simulink model "slo_flathier"  (R2015b)
settings: Solver=FixedStepDiscrete  SolverMode=SingleTasking  StartTime=0.0  StopTime=10  RelTol=1e-3
libraries: hdlsllib x1
CloseFcn:
  | rtwprivate ssgencode ModelCloseRequest Hysteresis_test1
settings Model: Creator=at-mt  LastModifiedBy=amatsumo
settings DataIOCC: SaveFormat=Array  SignalLoggingSaveFormat=ModelDataLogs  SaveOutput=off  SignalLogging=off  SaveTime=off
settings OptimizationCC: BlockReduction=off  ConditionallyExecuteInputs=off  DefaultParameterBehavior=Inlined  ExpressionDepthLimit=2147483647
settings DebuggingCC: AlgebraicLoopMsg=error  UnderspecifiedInitializationDetection=Classic  MergeDetectMultiDrivingBlocksExec=none  SolverPrmCheckMsg=warning  SingleTaskRateTransMsg=error  FcnCallInpInsideContextMsg=UseLocalSettings  StateNameClashWarn=warning
settings HardwareCC: ProdBitPerPointer=32  ProdLargestAtomicFloat=None  ProdIntDivRoundTo=Undefined  ProdEndianess=Unspecified  ProdWordSize=32  ProdHWDeviceType=ASIC/FPGA->ASIC/FPGA  ProdEqTarget=off
settings GRTTargetCC: GeneratePreprocessorConditionals=Disable all  CombineOutputUpdateFcns=off  GRTInterface=on
settings ConfigComp: CovModelRefEnable=Off  CovSFcnEnable=off

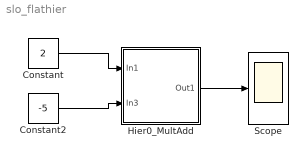
== system slo_flathier ==
  Constant : Constant  Value=2  OutDataTypeStr=int8
  Constant2 : Constant  Value=-5  OutDataTypeStr=int8
  Hier0_MultAdd : Subsystem
  Scope : Scope
  wires:
  Constant/1 -> Hier0_MultAdd/1(In1)
  Constant2/1 -> Hier0_MultAdd/2(In3)
  Hier0_MultAdd/1(Out1) -> Scope/1

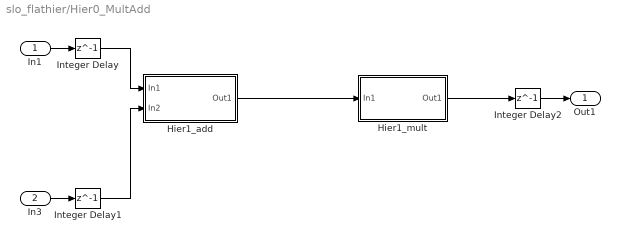
== system slo_flathier/Hier0_MultAdd ==
  In1 : Inport
  In3 : Inport  Port=2
  Hier1_add : Subsystem
  Hier1_mult : Subsystem
  Integer Delay : Delay  DelayLength=1  InputProcessing=Inherited
  Integer Delay1 : Delay  DelayLength=1  InputProcessing=Inherited
  Integer Delay2 : Delay  DelayLength=1  InputProcessing=Inherited
  Out1 : Outport
  wires:
  In1/1 -> Integer Delay/1
  Hier1_mult/1(Out1) -> Integer Delay2/1
  In3/1 -> Integer Delay1/1
  Hier1_add/1(Out1) -> Hier1_mult/1(In1)
  Integer Delay/1 -> Hier1_add/1(In1)
  Integer Delay1/1 -> Hier1_add/2(In2)
  Integer Delay2/1 -> Out1/1

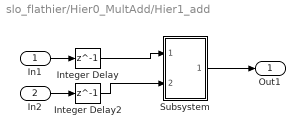
== system slo_flathier/Hier0_MultAdd/Hier1_add ==
  In1 : Inport
  In2 : Inport  Port=2
  Integer Delay : Delay  DelayLength=1  InputProcessing=Inherited
  Integer Delay2 : Delay  DelayLength=1  InputProcessing=Inherited
  Subsystem : Subsystem
  Out1 : Outport
  wires:
  Integer Delay/1 -> Subsystem/1(In1)
  Integer Delay2/1 -> Subsystem/2(In2)
  In1/1 -> Integer Delay/1
  Subsystem/1(Out1) -> Out1/1
  In2/1 -> Integer Delay2/1

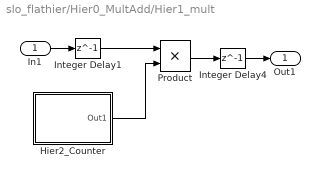
== system slo_flathier/Hier0_MultAdd/Hier1_mult ==
  In1 : Inport
  Hier2_Counter : Subsystem
  Integer Delay1 : Delay  DelayLength=1  InputProcessing=Inherited
  Integer Delay4 : Delay  DelayLength=1  InputProcessing=Inherited
  Product : Product  RndMeth=Zero
  Out1 : Outport
  wires:
  Product/1 -> Integer Delay4/1
  Integer Delay1/1 -> Product/1
  In1/1 -> Integer Delay1/1
  Integer Delay4/1 -> Out1/1
  Hier2_Counter/1(Out1) -> Product/2

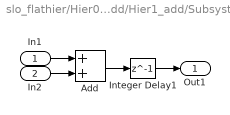
== system slo_flathier/Hier0_MultAdd/Hier1_add/Subsystem ==
  In1 : Inport
  In2 : Inport  Port=2
  Add : Sum
  Integer Delay1 : Delay  DelayLength=1  InputProcessing=Inherited
  Out1 : Outport
  wires:
  Add/1 -> Integer Delay1/1
  In1/1 -> Add/1
  Integer Delay1/1 -> Out1/1
  In2/1 -> Add/2

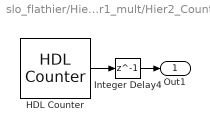
== system slo_flathier/Hier0_MultAdd/Hier1_mult/Hier2_Counter ==
  HDL Counter : hdlsllib/HDL Operations/HDL Counter  CountType=Free running  CountInit=0  CountStep=1  CountMax=100  CountFromType=Initial value  CountFrom=0  CountResetPort=off  CountLoadPort=off  CountEnbPort=off  CountDirPort=off  CountDataType=Unsigned  CountWordLen=3  CountFracLen=0  CountSampTime=1
  Integer Delay4 : Delay  DelayLength=1  InputProcessing=Inherited
  Out1 : Outport
  wires:
  HDL Counter/1 -> Integer Delay4/1
  Integer Delay4/1 -> Out1/1
